simulink model "ASDdc"  (R2018a)
settings: configuration reference "cs_ert" (kept outside this file)
settings Model: DataDictionary=ASDdc.sldd  Creator=zhoutinglin  LastModifiedBy=zhoutinglin

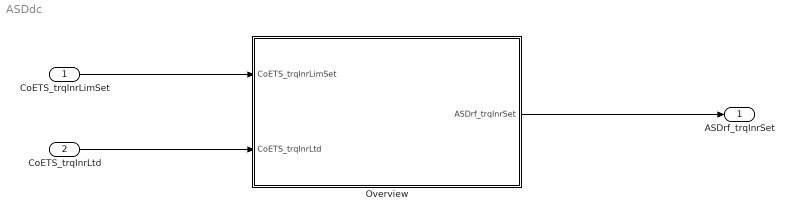
== system ASDdc ==
  CoETS_trqInrLimSet : Inport
  CoETS_trqInrLtd : Inport  Port=2
  Overview : Subsystem
  ASDrf_trqInrSet : Outport
  wires:
  CoETS_trqInrLimSet/1 -> Overview/1(CoETS_trqInrLimSet)
  CoETS_trqInrLtd/1 -> Overview/2(CoETS_trqInrLtd)
  Overview/1(ASDrf_trqInrSet) -> ASDrf_trqInrSet/1

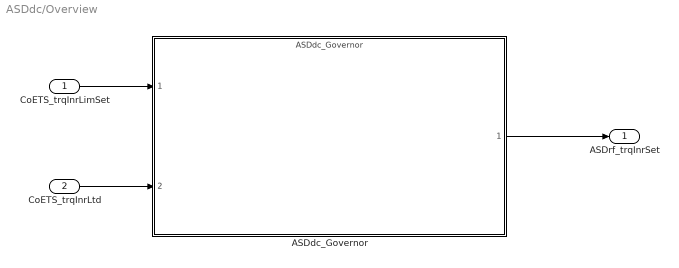
== system ASDdc/Overview ==
  CoETS_trqInrLimSet : Inport
  CoETS_trqInrLtd : Inport  Port=2
  ASDdc_Governor : ModelReference  ModelNameDialog=ASDdc_Governor  SimulationMode=Normal  ModelReferenceVersion=1.52
  ASDrf_trqInrSet : Outport
  wires:
  CoETS_trqInrLimSet/1 -> ASDdc_Governor/1
  CoETS_trqInrLtd/1 -> ASDdc_Governor/2
  ASDdc_Governor/1 -> ASDrf_trqInrSet/1
